simulink model "inlamningregler22"  (R2015a)
settings: Solver=ode45  StartTime=0.0  StopTime=2500  RelTol=1e-3
settings Model: Creator=mikpau  LastModifiedBy=mikpau

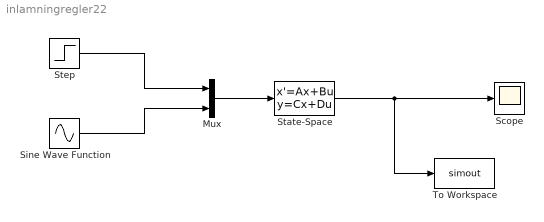
== system inlamningregler22 ==
  Mux : Mux  Inputs=2
  Scope : Scope
  Sine Wave Function : Sin  TimeSource=Use external signal  SampleTime=0
  State-Space : StateSpace  A=[-10/2000 3/2000; 3/1536 -3/1536]  B=[1/2000 7/2000; 0 0]  C=[1 0; 0 1]  D=[0 0; 0 0]  X0=0
  Step : Step  After=2500  SampleTime=0
  To Workspace : ToWorkspace  VariableName=simout  SaveFormat=Timeseries  SampleTime=-1
  wires:
  Mux/1 -> State-Space/1
  Step/1 -> Mux/1
  Sine Wave Function/1 -> Mux/2
  State-Space/1 -> To Workspace/1, Scope/1
